simulink model "PoseSimulation"  (R2023b)
settings: Solver=VariableStepAuto  StartTime=0.0  StopTime=simtime  RelTol=1e-3
values from neighbouring files (symbols this model uses):
  f_level = 2    [Fucntions_Test.m]    (also in Functions_Test.m)
  f_max = 100    [Fucntions_Test.m]    (also in Functions_Test.m = 10)
  f_min = 10    [Fucntions_Test.m]    (also in Functions_Test.m = 1)
  Kd = diag([3 3 1])    [PoseSimulationScript.m]
  Ki = diag([3 3 3])    [PoseSimulationScript.m]
  Kp = diag([8 8 4])    [PoseSimulationScript.m]
  y_0 = [0,0,0]'    [PoseSimulationScript.m]
  y_reference = [0.4,-0.4,deg2rad(20)]'    [PoseSimulationScript.m]
undefined symbols (not defined in the file or in its folder): a, b, Iz, m, Wp
settings Model: Creator=eliasoa  LastModifiedBy=eliasoa

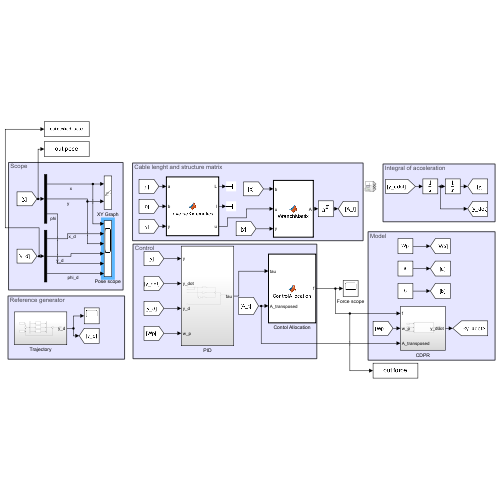
[thumbnail: Simulink's stored preview of the top-level diagram]
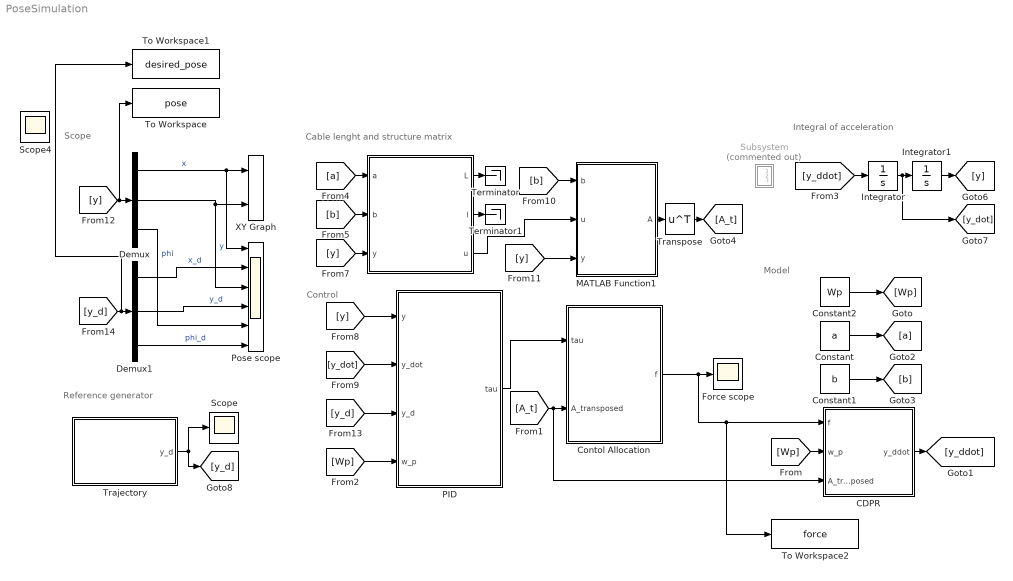
== system PoseSimulation ==
  note: Cable lenght and structure matrix
  note: Reference generator
  note: Model
  note: Control
  note: Integral of acceleration
  note: Scope
  " " : MATLAB Function  TreatAsAtomicUnit=on
  CDPR : Subsystem
  Constant : Constant  Value=a
  Constant1 : Constant  Value=b
  Constant2 : Constant  Value=Wp
  Contol Allocation : MATLAB Function  TreatAsAtomicUnit=on
  Demux : Demux  Outputs=3
  Demux1 : Demux  Outputs=3
  Force scope : Scope
  Integrator : Integrator  InitialCondition=[0; 0; 0];
  Integrator1 : Integrator  InitialCondition=y_0
  MATLAB Function1 : MATLAB Function  TreatAsAtomicUnit=on
  "PID " : Subsystem
  Pose scope : Scope  NumInputPorts=6
  Scope : Scope
  Subsystem : Subsystem  Commented=on
  Terminator : Terminator
  Terminator1 : Terminator
  To Workspace : ToWorkspace  VariableName=pose  SaveFormat=Timeseries  SampleTime=-1
  To Workspace1 : ToWorkspace  VariableName=desired_pose  SaveFormat=Timeseries  SampleTime=-1
  To Workspace2 : ToWorkspace  VariableName=force  SaveFormat=Timeseries  SampleTime=-1
  Trajectory : Subsystem
  Transpose : Math  Operator=transpose
  XY Graph : Record  FileSettingsInternal="{\"entries\":[{\"content\":{\"excelSettings\":{\"content\":{},\"type\":\"Streamout.ExcelSettings\"}},\"type\":\"Streamout.FileSettingStorage\",\"uuid\":\"\"}],\"packageUris\":[\"http:\\/\\/schema.mathworks.com\\/mf0\\/streamout_blocks\\/R2020a\"],\"version\":\"1.0\"}"  Layout=[1 1]  SignalsInternal="{\"entries\":[{\"content\":{\"signals\":[{\"content\":{\"blockPath\":[],\"dimensions\":[1,1],\"domain\":\"\",\"lineColor\":\"#4dbeee\",\"plots\":[1],\"port\":1,\"sid\":[\"\"],\"signalID\":1641,\"signalName\":\"x\"},\"type\":\"RecordBlkView.Signal\",\"uuid\":\"\"},{\"content\":{\"blockPath\":[],\"dimensions\":[1,1],\"domain\":\"\",\"lineColor\":\"#a2142f\",\"plots\":[1],\"port\":2,\"sid\":[\"\"],\"signalID\":1645,\"signalName\":\"y\"},\"type\":\"RecordBlkView.Signal\",\"uuid\":\"\"}]},\"type\":\"RecordBlkView.InputSignals\",\"uuid\":\"\"}],\"packageUris\":[\"http:\\/\\/schema.mathworks.com\\/mf0\\/streamout_blocks\\/R2020a\"],\"version\":\"1.0\"}"  VisualizationBindings="{\"xyplotplugin\":{\"info\":[{\"series\":[{\"bindingParametersList\":[{\"parameter\":\"X-Axis\",\"signalID\":1641,\"signalName\":\"x\"},{\"parameter\":\"Y-Axis\",\"signalID\":1645,\"signalName\":\"y\"}],\"seriesID\":21925}],\"subplotID\":1}]}}"  CompatibilityTag=XY
  Scope4 : Scope
  wires:
  "PID "/1(tau) -> Contol Allocation/1(tau)
  Contol Allocation/1(f) -> To Workspace2/1, CDPR/1(f), Force scope/1
  [A_t] -> CDPR/3(A_transposed), Contol Allocation/2(A_transposed)
  Integrator/1 -> [y_dot], Integrator1/1
  CDPR/1(y_ddot) -> [y_ddot]
  Constant2/1 -> [Wp]
  [Wp] -> CDPR/2(w_p)
  [Wp] -> "PID "/4(w_p)
  [y_ddot] -> Integrator/1
  Constant1/1 -> [b]
  Constant/1 -> [a]
  [b] -> " "/2(b)
  [a] -> " "/1(a)
  MATLAB Function1/1(A) -> Transpose/1
  Transpose/1 -> [A_t]
  " "/3(u) -> MATLAB Function1/2(u)
  [y] -> " "/3(y)
  Integrator1/1 -> [y]
  [y] -> "PID "/1(y)
  [y_dot] -> "PID "/2(y_dot)
  [b] -> MATLAB Function1/1(b)
  [y] -> MATLAB Function1/3(y)
  [y_d] -> "PID "/3(y_d)
  Trajectory/1(y_d) -> [y_d], Scope/1
  Demux1/3 -> Pose scope/6  "phi_d"
  Demux1/2 -> Pose scope/4  "y_d"
  Demux1/1 -> Pose scope/2  "x_d"
  Demux/3 -> Pose scope/5  "phi"
  Demux/2 -> XY Graph/2, Pose scope/3  "y"
  Demux/1 -> XY Graph/1, Pose scope/1  "x"
  [y] -> To Workspace/1, Demux/1
  [y_d] -> To Workspace1/1, Demux1/1
  " "/2(l) -> Terminator1/1
  " "/1(L) -> Terminator/1

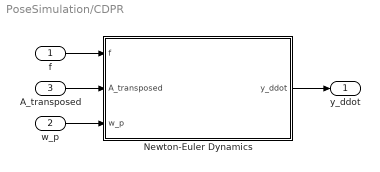
== system PoseSimulation/CDPR ==
  f : Inport
  w_p : Inport  Port=2
  A_transposed : Inport  Port=3
  "Newton-Euler Dynamics " : Subsystem
  y_ddot : Outport
  wires:
  "Newton-Euler Dynamics "/1(y_ddot) -> y_ddot/1
  A_transposed/1 -> "Newton-Euler Dynamics "/2(A_transposed)
  f/1 -> "Newton-Euler Dynamics "/1(f)
  w_p/1 -> "Newton-Euler Dynamics "/3(w_p)

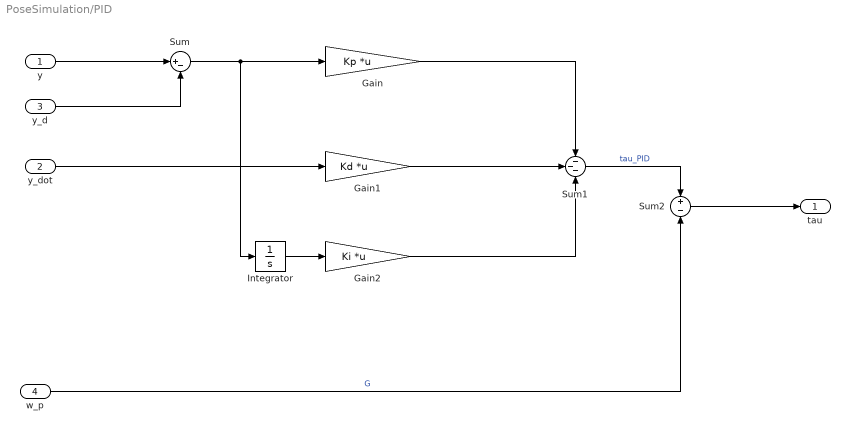
== system PoseSimulation/PID  ==
  y : Inport
  y_dot : Inport  Port=2
  y_d : Inport  Port=3
  w_p : Inport  Port=4
  Gain : Gain  Gain=Kp  Multiplication=Matrix(K*u)
  Gain1 : Gain  Gain=Kd  Multiplication=Matrix(K*u)
  Gain2 : Gain  Gain=Ki  Multiplication=Matrix(K*u)
  Integrator : Integrator
  Sum : Sum  Inputs=|+-
  Sum1 : Sum  Inputs=---
  Sum2 : Sum  Inputs=+|-
  tau : Outport
  wires:
  y/1 -> Sum/1
  y_d/1 -> Sum/2
  Sum/1 -> Integrator/1, Gain/1
  y_dot/1 -> Gain1/1
  Sum2/1 -> tau/1
  w_p/1 -> Sum2/2  "G"
  Gain1/1 -> Sum1/2
  Gain/1 -> Sum1/1
  Integrator/1 -> Gain2/1
  Gain2/1 -> Sum1/3
  Sum1/1 -> Sum2/1  "tau_PID"

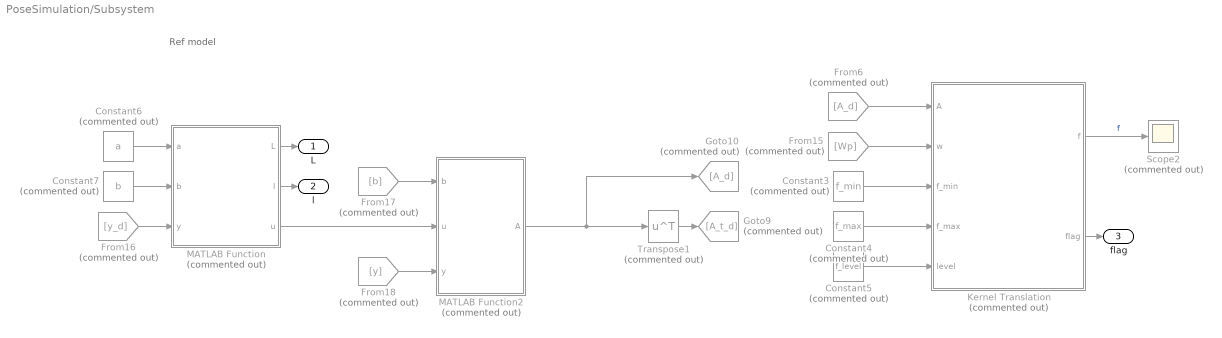
== system PoseSimulation/Subsystem ==
  note: Ref model
  Constant3 : Constant  Commented=on  Value=f_min
  Constant4 : Constant  Commented=on  Value=f_max
  Constant5 : Constant  Commented=on  Value=f_level
  Constant6 : Constant  Commented=on  Value=a
  Constant7 : Constant  Commented=on  Value=b
  From15 : From  Commented=on  GotoTag=Wp
  From16 : From  Commented=on  GotoTag=y_d
  From17 : From  Commented=on  GotoTag=b
  From18 : From  Commented=on  GotoTag=y
  From6 : From  Commented=on  GotoTag=A_d
  Goto10 : Goto  Commented=on  GotoTag=A_d
  Goto9 : Goto  Commented=on  GotoTag=A_t_d
  Kernel Translation : MATLAB Function  Commented=on  TreatAsAtomicUnit=on
  MATLAB Function : MATLAB Function  Commented=on  TreatAsAtomicUnit=on
  MATLAB Function2 : MATLAB Function  Commented=on  TreatAsAtomicUnit=on
  Scope2 : Scope  Commented=on
  Transpose1 : Math  Commented=on  Operator=transpose
  L : Outport
  l : Outport  Port=2
  flag : Outport  Port=3
  wires:
  Constant7/1 -> MATLAB Function/2(b)
  Kernel Translation/2(flag) -> flag/1
  From17/1 -> MATLAB Function2/1(b)
  From18/1 -> MATLAB Function2/3(y)
  MATLAB Function2/1(A) -> Goto10/1, Transpose1/1
  MATLAB Function/3(u) -> MATLAB Function2/2(u)
  Constant3/1 -> Kernel Translation/3(f_min)
  Transpose1/1 -> Goto9/1
  From16/1 -> MATLAB Function/3(y)
  Constant6/1 -> MATLAB Function/1(a)
  From15/1 -> Kernel Translation/2(w)
  From6/1 -> Kernel Translation/1(A)
  Kernel Translation/1(f) -> Scope2/1  "f"
  MATLAB Function/2(l) -> l/1
  Constant5/1 -> Kernel Translation/5(level)
  Constant4/1 -> Kernel Translation/4(f_max)
  MATLAB Function/1(L) -> L/1

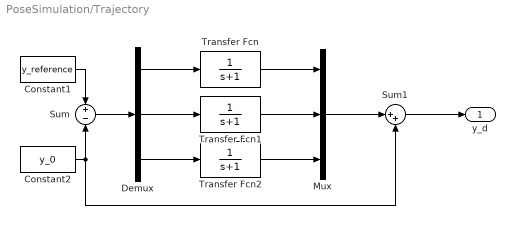
== system PoseSimulation/Trajectory ==
  Constant1 : Constant  Value=y_reference
  Constant2 : Constant  Value=y_0
  Demux : Demux  Outputs=3
  Mux : Mux  Inputs=3
  Sum : Sum  Inputs=+-
  Sum1 : Sum  Inputs=|++
  Transfer Fcn : TransferFcn  Denominator=[1 1]
  Transfer Fcn1 : TransferFcn  Denominator=[1 1]
  Transfer Fcn2 : TransferFcn  Denominator=[1 1]
  y_d : Outport
  wires:
  Transfer Fcn2/1 -> Mux/3
  Transfer Fcn1/1 -> Mux/2
  Transfer Fcn/1 -> Mux/1
  Demux/2 -> Transfer Fcn1/1
  Demux/1 -> Transfer Fcn/1
  Demux/3 -> Transfer Fcn2/1
  Constant1/1 -> Sum/1
  Mux/1 -> Sum1/1
  Sum1/1 -> y_d/1
  Sum/1 -> Demux/1
  Constant2/1 -> Sum1/2, Sum/2

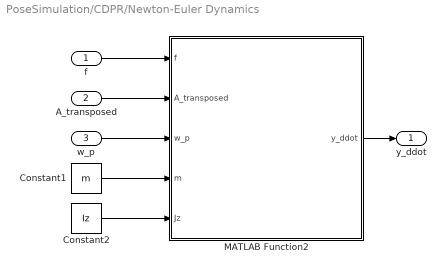
== system PoseSimulation/CDPR/Newton-Euler Dynamics  ==
  f : Inport
  A_transposed : Inport  Port=2
  w_p : Inport  Port=3
  Constant1 : Constant  Value=m
  Constant2 : Constant  Value=Iz
  MATLAB Function2 : MATLAB Function  TreatAsAtomicUnit=on
  y_ddot : Outport
  wires:
  MATLAB Function2/1(y_ddot) -> y_ddot/1
  f/1 -> MATLAB Function2/1(f)
  A_transposed/1 -> MATLAB Function2/2(A_transposed)
  Constant1/1 -> MATLAB Function2/4(m)
  Constant2/1 -> MATLAB Function2/5(Jz)
  w_p/1 -> MATLAB Function2/3(w_p)

== matlab function PoseSimulation/MATLAB Function1 ==
  data: b input; u input; A output; y input
function A = WrenchMatrix(b, u, y)
    A = WrenchMatrix(b, u, y);
end

== matlab function PoseSimulation/  ==
  data: a input; L output; b input; y input; l output; u output
function [L,l,u] = InverseKinematics(a, b, y)
    [L,l,u] = InverseKinematics(a, b, y);
end

== matlab function PoseSimulation/Subsystem/MATLAB Function ==
  data: a input; L output; b input; y input; l output; u output
function [L,l,u] = InverseKinematics(a, b, y)
    [L,l,u] = InverseKinematics(a, b, y);
end

== matlab function PoseSimulation/Contol Allocation ==
  data: tau input; f output; A_transposed input
function f = ControlAllocation(tau, A_transposed)
A_PseudoInv = A_transposed'/(A_transposed*A_transposed');
f = A_PseudoInv*tau;
end

== matlab function PoseSimulation/CDPR/Newton-Euler Dynamics /MATLAB Function2 ==
  data: y_ddot output; f input; A_transposed input; w_p input; m input; Jz input
function y_ddot = NewtonEuler_Dynamics(f, A_transposed, w_p, m, Jz)

y_ddot = CDPR_NewtonEuler_Dynamics(f, A_transposed, w_p, m, Jz);

== matlab function PoseSimulation/Subsystem/Kernel Translation ==
  data: A input; f output; w input; f_min input; f_max input; level input; flag output
function [f, flag] = Kernel_translation(A,w,f_min,f_max,level)
[f, flag] = Kernel_translation(A,w,f_min,f_max,level);
end

== matlab function PoseSimulation/Subsystem/MATLAB Function2 ==
  data: b input; u input; A output; y input
function A = WrenchMatrix(b, u, y)
    A = WrenchMatrix(b, u, y);
end
